simulink subsystem "Circuit_CT_SS"  (R2022a)
settings: Solver=VariableStepAuto  StartTime=0.0  StopTime=10.0  RelTol=1e-3
values from neighbouring files (symbols this model uses):
  C = eye(3)    [DAE_Circuit_main.m]
undefined symbols (not defined in the file or in its folder): A_CT, B_CT, x0
settings Model: Creator=tyevans  LastModifiedBy=tyevans

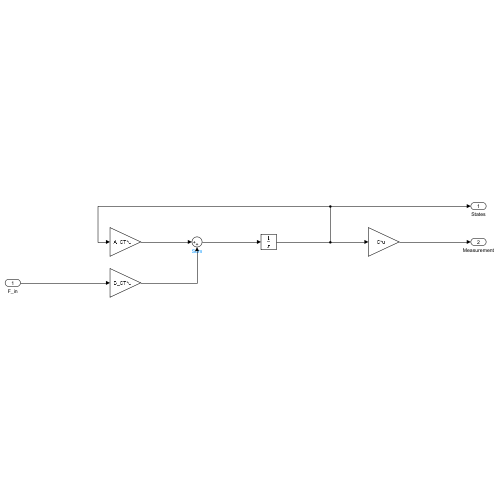
[thumbnail: Simulink's stored preview of the top-level diagram]
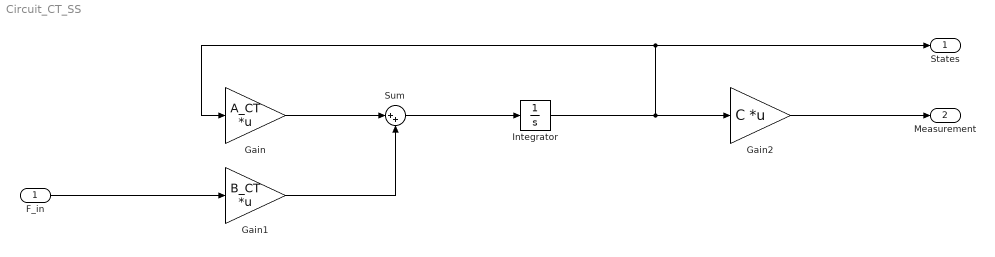
== system Circuit_CT_SS ==
  F_in : Inport
  Gain : Gain  Gain=A_CT  Multiplication=Matrix(K*u)
  Gain1 : Gain  Gain=B_CT  Multiplication=Matrix(K*u)
  Gain2 : Gain  Gain=C  Multiplication=Matrix(K*u)
  Integrator : Integrator  InitialCondition=x0
  Sum : Sum  Inputs=|++
  States : Outport
  Measurement : Outport  Port=2
  wires:
  Integrator/1 -> Gain2/1, Gain/1, States/1
  Gain2/1 -> Measurement/1
  F_in/1 -> Gain1/1
  Gain/1 -> Sum/1
  Sum/1 -> Integrator/1
  Gain1/1 -> Sum/2
